simulink model "synchronized"  (R2018b)
settings: Solver=FixedStepAuto  StartTime=0.0  StopTime=0.1  FixedStep=0.0001  RelTol=1e-3
settings Model: Creator=User  LastModifiedBy=User

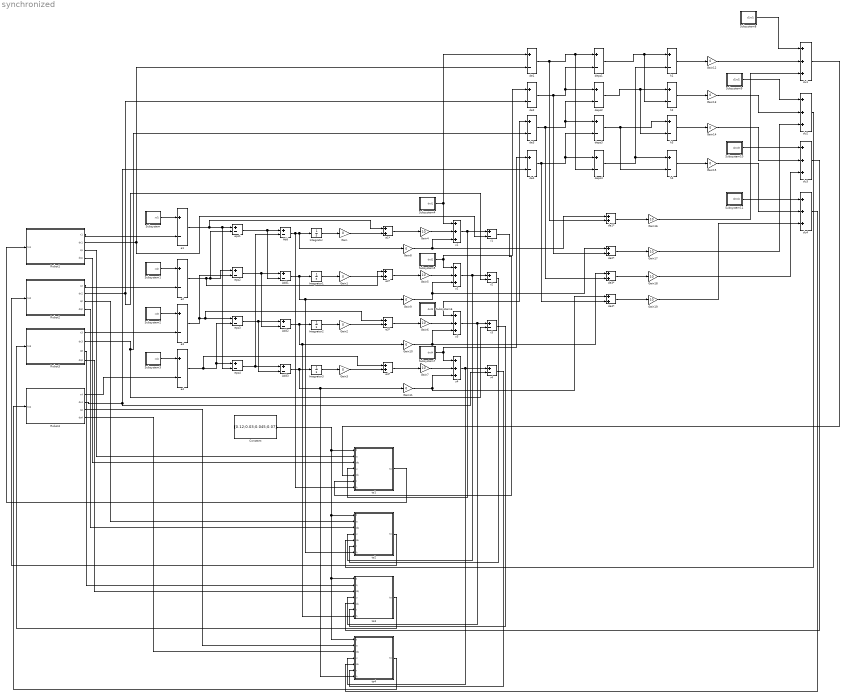
== system synchronized ==
  Add{,1..3} (4 alike) : Sum  Inputs=+-
  Constant : Constant  Value=[0.12;0.03;0.045;0.07]
  Gain{,1..3,8..15} (12 alike) : Gain  Gain=0
  Gain{4..7,16..19} (8 alike) : Gain  Gain=10
  Integrator{,1..3} (4 alike) : Integrator  InitialCondition=[0;0]
  Robot1 : Subsystem
  Robot2 : Subsystem
  Robot3 : Subsystem
  Robot4 : Subsystem
  Subsystem : Subsystem
  Subsystem1 : Subsystem
  Subsystem10 : Subsystem
  Subsystem11 : Subsystem
  Subsystem2 : Subsystem
  Subsystem3 : Subsystem
  Subsystem4 : Subsystem
  Subsystem5 : Subsystem
  Subsystem6 : Subsystem
  Subsystem7 : Subsystem
  Subsystem8 : Subsystem
  Subsystem9 : Subsystem
  de{1..4} (4 alike) : Sum  Inputs=+-
  de1* : Sum
  de2* : Sum
  de3* : Sum
  de4* : Sum
  deps{1..4} (4 alike) : Sum  Inputs=+-
  du{1..4} (4 alike) : Sum  Inputs=3
  e{1..4} (4 alike) : Sum  Inputs=+-
  e1* : Sum
  e2* : Sum
  e3* : Sum
  e4* : Sum
  eps{1..4} (4 alike) : Sum  Inputs=+-
  h{1..4} (4 alike) : Sum  Inputs=+-
  r{1..4} (4 alike) : Sum  Inputs=+-
  to1 : MATLAB Function  TreatAsAtomicUnit=on
  to2 : MATLAB Function  TreatAsAtomicUnit=on
  to3 : MATLAB Function  TreatAsAtomicUnit=on
  to4 : MATLAB Function  TreatAsAtomicUnit=on
  u{1..4} (4 alike) : Sum  Inputs=+++
  wires:
  Subsystem/1(xd1) -> e1/1
  Robot1/1(x1) -> e1/2
  Subsystem1/1(xd2) -> e2/1
  Robot2/1(x2) -> e2/2
  Robot3/1(x3) -> e3/2
  Subsystem2/1(xd3) -> e3/1
  Subsystem3/1(xd4) -> e4/1
  Robot4/1(x4) -> e4/2
  e1/1 -> e1*/1, eps4/2, eps1/1
  e2/1 -> e2*/1, eps1/2, eps2/1
  e3/1 -> e3*/1, eps3/1, eps2/2
  e4/1 -> e4*/1, eps4/1, eps3/2
  eps1/1 -> Add1/2, Add/1
  eps2/1 -> Add2/2, Add1/1
  eps3/1 -> Add2/1, Add3/2
  eps4/1 -> Add3/1, Add/2
  Add3/1 -> to4/7(h), Gain11/1, Integrator3/1
  Add2/1 -> to3/7(h), Gain10/1, Integrator2/1
  Add1/1 -> to2/7(h), Gain9/1, Integrator1/1
  Integrator/1 -> Gain/1
  Integrator1/1 -> Gain1/1
  Integrator2/1 -> Gain2/1
  Integrator3/1 -> Gain3/1
  Gain/1 -> e1*/2
  Gain1/1 -> e2*/2
  Gain2/1 -> e3*/2
  Gain3/1 -> e4*/2
  e1*/1 -> Gain4/1
  e4*/1 -> Gain7/1
  e3*/1 -> Gain6/1
  e2*/1 -> Gain5/1
  Subsystem4/1(dxd1) -> de1/1, u1/1
  Gain4/1 -> u1/2
  Gain8/1 -> de1*/1, u1/3
  Gain9/1 -> de2*/1, u2/3
  Gain5/1 -> u2/2
  Gain6/1 -> u3/2
  Gain10/1 -> de3*/1, u3/3
  Gain11/1 -> de4*/1, u4/3
  Gain7/1 -> u4/2
  Subsystem5/1(dxd2) -> de2/1, u2/1
  Subsystem6/1(dxd3) -> de3/1, u3/1
  Subsystem7/1(dxd4) -> de4/1, u4/1
  u4/1 -> to4/4(u), r4/1
  u3/1 -> to3/4(u), r3/1
  u2/1 -> to2/4(u), r2/1
  u1/1 -> to1/4(u), r1/1
  Robot1/2(dx1) -> r1/2, de1/2
  Robot2/2(dx2) -> r2/2, de2/2
  Robot3/2(dx3) -> de3/2, r3/2
  Robot4/2(dx4) -> de4/2, r4/2
  de1/1 -> de1*/2, deps4/2, deps1/1
  de2/1 -> de2*/2, deps2/1, deps1/2
  de3/1 -> de3*/2, deps3/1, deps2/2
  de4/1 -> de4*/2, deps4/1, deps3/2
  deps1/1 -> h2/2, h1/1
  deps4/1 -> h4/1, h1/2
  deps2/1 -> h3/2, h2/1
  deps3/1 -> h4/2, h3/1
  h1/1 -> Gain12/1
  h2/1 -> Gain13/1
  h3/1 -> Gain14/1
  h4/1 -> Gain15/1
  Gain12/1 -> du1/2
  Gain13/1 -> du2/2
  Gain14/1 -> du3/2
  Gain15/1 -> du4/2
  Subsystem8/1(d2xd1) -> du1/1
  Subsystem9/1(d2xd2) -> du2/1
  Subsystem10/1(d2xd3) -> du3/1
  Subsystem11/1(d2xd4) -> du4/1
  de4*/1 -> Gain19/1
  de3*/1 -> Gain18/1
  de2*/1 -> Gain17/1
  de1*/1 -> Gain16/1
  Gain16/1 -> du1/3
  Gain17/1 -> du2/3
  Gain18/1 -> du3/3
  Gain19/1 -> du4/3
  Robot1/3(q1) -> to1/2(q)
  Robot1/4(dq1) -> to1/3(dq)
  du1/1 -> to1/5(du)
  r1/1 -> to1/6(r)
  Add/1 -> to1/7(h), Gain8/1, Integrator/1
  Robot2/3(q2) -> to2/2(q)
  Robot2/4(dq2) -> to2/3(dq)
  Robot3/3(q3) -> to3/2(q)
  Robot3/4(dq3) -> to3/3(dq)
  Robot4/3(q4) -> to4/2(q)
  Robot4/4(dq4) -> to4/3(dq)
  r2/1 -> to2/6(r)
  r3/1 -> to3/6(r)
  r4/1 -> to4/6(r)
  du2/1 -> to2/5(du)
  du3/1 -> to3/5(du)
  du4/1 -> to4/5(du)
  to1/1(to) -> Robot1/1(to1)
  to2/1(to) -> Robot2/1(to2)
  to3/1(to) -> Robot3/1(to3)
  to4/1(to) -> Robot4/1(to4)
  Constant/1 -> to4/1(t), to3/1(t), to2/1(t), to1/1(t)

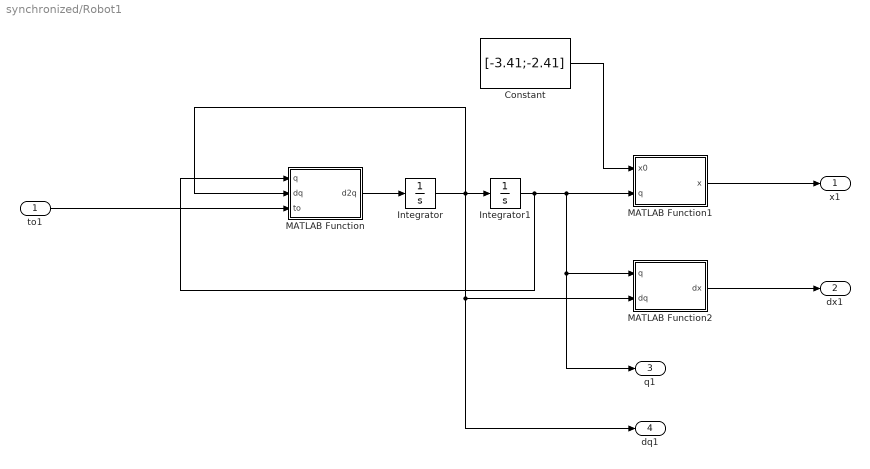
== system synchronized/Robot1 ==
  to1 : Inport
  Constant : Constant  Value=[-3.41;-2.41]
  Integrator : Integrator  InitialCondition=[0;0]
  Integrator1 : Integrator  InitialCondition=[pi/6;pi/6]
  MATLAB Function : MATLAB Function  TreatAsAtomicUnit=on
  MATLAB Function1 : MATLAB Function  TreatAsAtomicUnit=on
  MATLAB Function2 : MATLAB Function  TreatAsAtomicUnit=on
  x1 : Outport
  dx1 : Outport  Port=2
  q1 : Outport  Port=3
  dq1 : Outport  Port=4
  wires:
  to1/1 -> MATLAB Function/3(to)
  MATLAB Function/1(d2q) -> Integrator/1
  Integrator/1 -> dq1/1, MATLAB Function2/2(dq), MATLAB Function/2(dq), Integrator1/1
  Integrator1/1 -> q1/1, MATLAB Function2/1(q), MATLAB Function1/2(q), MATLAB Function/1(q)
  MATLAB Function1/1(x) -> x1/1
  Constant/1 -> MATLAB Function1/1(x0)
  MATLAB Function2/1(dx) -> dx1/1

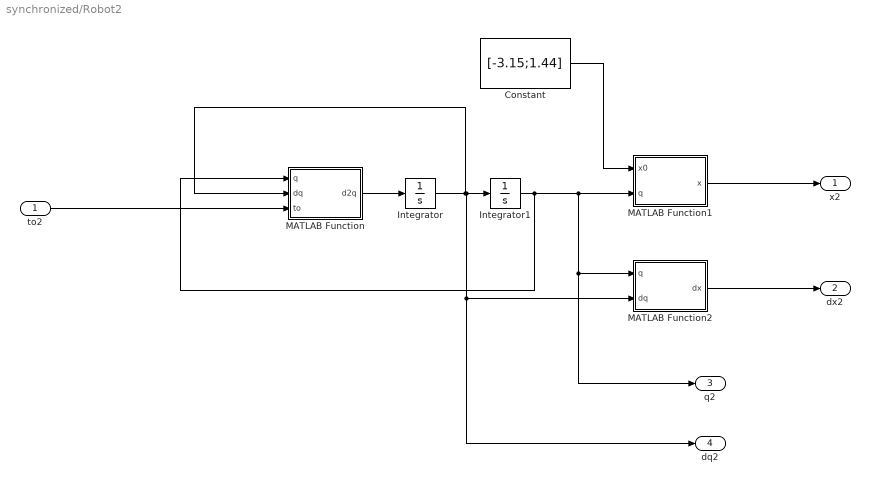
== system synchronized/Robot2 ==
  to2 : Inport
  Constant : Constant  Value=[-3.15;1.44]
  Integrator : Integrator  InitialCondition=[0;0]
  Integrator1 : Integrator  InitialCondition=[-0.37895;2.3932]
  MATLAB Function : MATLAB Function  TreatAsAtomicUnit=on
  MATLAB Function1 : MATLAB Function  TreatAsAtomicUnit=on
  MATLAB Function2 : MATLAB Function  TreatAsAtomicUnit=on
  x2 : Outport
  dx2 : Outport  Port=2
  q2 : Outport  Port=3
  dq2 : Outport  Port=4
  wires:
  Constant/1 -> MATLAB Function1/1(x0)
  MATLAB Function1/1(x) -> x2/1
  Integrator1/1 -> MATLAB Function/1(q), q2/1, MATLAB Function2/1(q), MATLAB Function1/2(q)
  Integrator/1 -> dq2/1, MATLAB Function2/2(dq), Integrator1/1, MATLAB Function/2(dq)
  MATLAB Function/1(d2q) -> Integrator/1
  to2/1 -> MATLAB Function/3(to)
  MATLAB Function2/1(dx) -> dx2/1

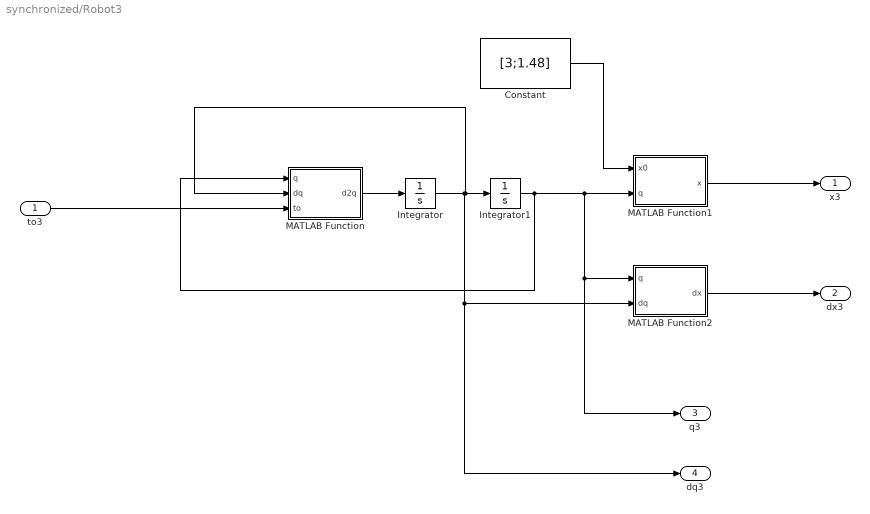
== system synchronized/Robot3 ==
  to3 : Inport
  Constant : Constant  Value=[3;1.48]
  Integrator : Integrator  InitialCondition=[0;0]
  Integrator1 : Integrator  InitialCondition=[-pi/6;pi/3]
  MATLAB Function : MATLAB Function  TreatAsAtomicUnit=on
  MATLAB Function1 : MATLAB Function  TreatAsAtomicUnit=on
  MATLAB Function2 : MATLAB Function  TreatAsAtomicUnit=on
  x3 : Outport
  dx3 : Outport  Port=2
  q3 : Outport  Port=3
  dq3 : Outport  Port=4
  wires:
  to3/1 -> MATLAB Function/3(to)
  MATLAB Function/1(d2q) -> Integrator/1
  Integrator/1 -> dq3/1, MATLAB Function2/2(dq), MATLAB Function/2(dq), Integrator1/1
  Integrator1/1 -> q3/1, MATLAB Function2/1(q), MATLAB Function1/2(q), MATLAB Function/1(q)
  MATLAB Function1/1(x) -> x3/1
  Constant/1 -> MATLAB Function1/1(x0)
  MATLAB Function2/1(dx) -> dx3/1

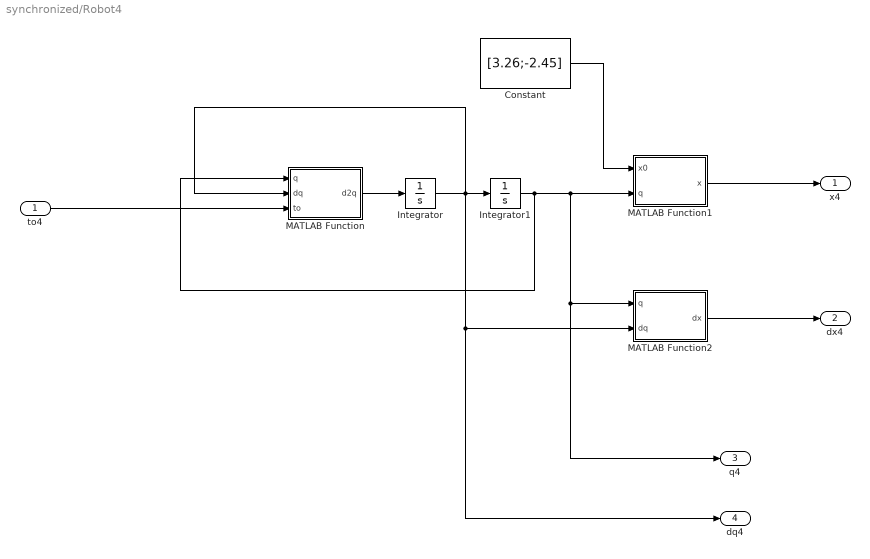
== system synchronized/Robot4 ==
  to4 : Inport
  Constant : Constant  Value=[3.26;-2.45]
  Integrator : Integrator  InitialCondition=[0;0]
  Integrator1 : Integrator  InitialCondition=[5*pi/6;-pi/3]
  MATLAB Function : MATLAB Function  TreatAsAtomicUnit=on
  MATLAB Function1 : MATLAB Function  TreatAsAtomicUnit=on
  MATLAB Function2 : MATLAB Function  TreatAsAtomicUnit=on
  x4 : Outport
  dx4 : Outport  Port=2
  q4 : Outport  Port=3
  dq4 : Outport  Port=4
  wires:
  Constant/1 -> MATLAB Function1/1(x0)
  MATLAB Function1/1(x) -> x4/1
  Integrator1/1 -> MATLAB Function/1(q), q4/1, MATLAB Function2/1(q), MATLAB Function1/2(q)
  Integrator/1 -> dq4/1, MATLAB Function2/2(dq), MATLAB Function/2(dq), Integrator1/1
  MATLAB Function/1(d2q) -> Integrator/1
  to4/1 -> MATLAB Function/3(to)
  MATLAB Function2/1(dx) -> dx4/1

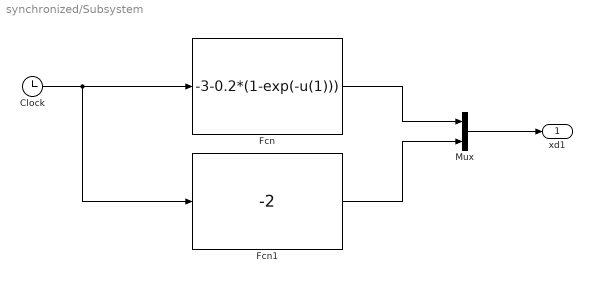
== system synchronized/Subsystem ==
  Clock : Clock
  Fcn : Fcn  Expr=-3-0.2*(1-exp(-u(1)))
  Fcn1 : Fcn  Expr=-2
  Mux : Mux  Inputs=2
  xd1 : Outport
  wires:
  Clock/1 -> Fcn1/1, Fcn/1
  Fcn/1 -> Mux/1
  Fcn1/1 -> Mux/2
  Mux/1 -> xd1/1

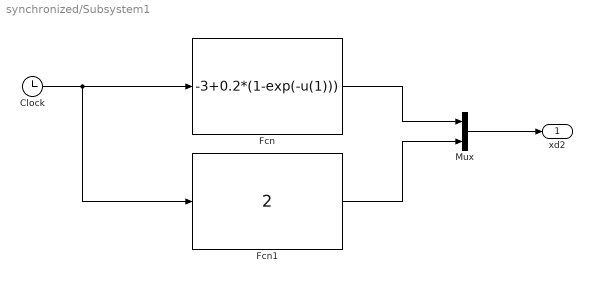
== system synchronized/Subsystem1 ==
  Clock : Clock
  Fcn : Fcn  Expr=-3+0.2*(1-exp(-u(1)))
  Fcn1 : Fcn  Expr=2
  Mux : Mux  Inputs=2
  xd2 : Outport
  wires:
  Mux/1 -> xd2/1
  Fcn1/1 -> Mux/2
  Fcn/1 -> Mux/1
  Clock/1 -> Fcn/1, Fcn1/1

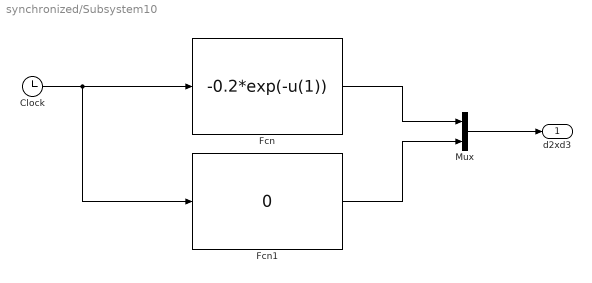
== system synchronized/Subsystem10 ==
  Clock : Clock
  Fcn : Fcn  Expr=-0.2*exp(-u(1))
  Fcn1 : Fcn  Expr=0
  Mux : Mux  Inputs=2
  d2xd3 : Outport
  wires:
  Clock/1 -> Fcn1/1, Fcn/1
  Fcn/1 -> Mux/1
  Fcn1/1 -> Mux/2
  Mux/1 -> d2xd3/1

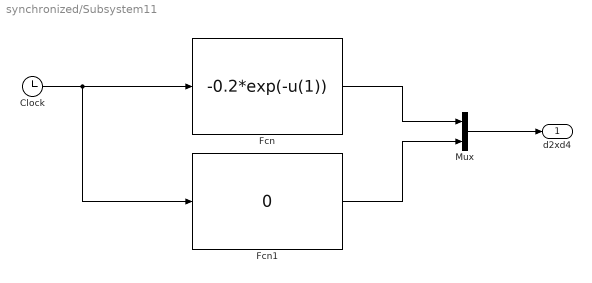
== system synchronized/Subsystem11 ==
  Clock : Clock
  Fcn : Fcn  Expr=-0.2*exp(-u(1))
  Fcn1 : Fcn  Expr=0
  Mux : Mux  Inputs=2
  d2xd4 : Outport
  wires:
  Mux/1 -> d2xd4/1
  Fcn1/1 -> Mux/2
  Fcn/1 -> Mux/1
  Clock/1 -> Fcn/1, Fcn1/1

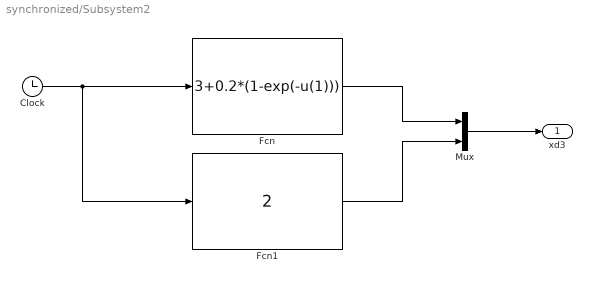
== system synchronized/Subsystem2 ==
  Clock : Clock
  Fcn : Fcn  Expr=3+0.2*(1-exp(-u(1)))
  Fcn1 : Fcn  Expr=2
  Mux : Mux  Inputs=2
  xd3 : Outport
  wires:
  Clock/1 -> Fcn1/1, Fcn/1
  Fcn/1 -> Mux/1
  Fcn1/1 -> Mux/2
  Mux/1 -> xd3/1

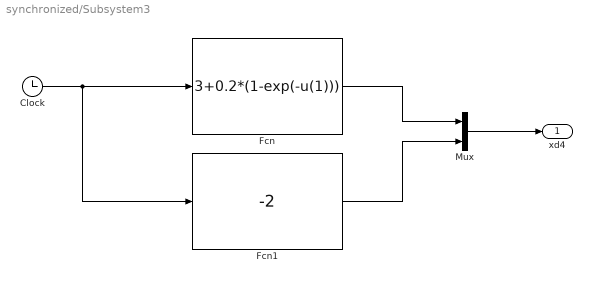
== system synchronized/Subsystem3 ==
  Clock : Clock
  Fcn : Fcn  Expr=3+0.2*(1-exp(-u(1)))
  Fcn1 : Fcn  Expr=-2
  Mux : Mux  Inputs=2
  xd4 : Outport
  wires:
  Mux/1 -> xd4/1
  Fcn1/1 -> Mux/2
  Fcn/1 -> Mux/1
  Clock/1 -> Fcn/1, Fcn1/1

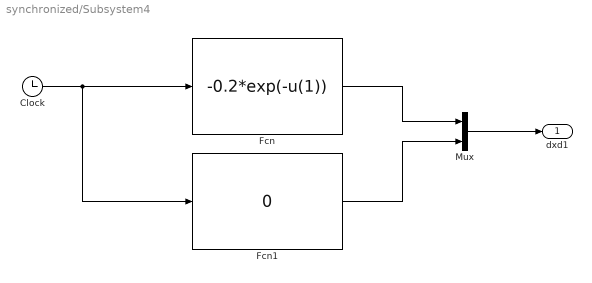
== system synchronized/Subsystem4 ==
  Clock : Clock
  Fcn : Fcn  Expr=-0.2*exp(-u(1))
  Fcn1 : Fcn  Expr=0
  Mux : Mux  Inputs=2
  dxd1 : Outport
  wires:
  Mux/1 -> dxd1/1
  Fcn1/1 -> Mux/2
  Fcn/1 -> Mux/1
  Clock/1 -> Fcn/1, Fcn1/1

== system synchronized/Subsystem5 ==
  Clock : Clock
  Fcn : Fcn  Expr=0.2*exp(-u(1))
  Fcn1 : Fcn  Expr=0
  Mux : Mux  Inputs=2
  dxd2 : Outport
  wires:
  Clock/1 -> Fcn1/1, Fcn/1
  Fcn/1 -> Mux/1
  Fcn1/1 -> Mux/2
  Mux/1 -> dxd2/1

== system synchronized/Subsystem6 ==
  Clock : Clock
  Fcn : Fcn  Expr=0.2*exp(-u(1))
  Fcn1 : Fcn  Expr=0
  Mux : Mux  Inputs=2
  dxd3 : Outport
  wires:
  Mux/1 -> dxd3/1
  Fcn1/1 -> Mux/2
  Fcn/1 -> Mux/1
  Clock/1 -> Fcn/1, Fcn1/1

== system synchronized/Subsystem7 ==
  Clock : Clock
  Fcn : Fcn  Expr=0.2*exp(-u(1))
  Fcn1 : Fcn  Expr=0
  Mux : Mux  Inputs=2
  dxd4 : Outport
  wires:
  Clock/1 -> Fcn1/1, Fcn/1
  Fcn/1 -> Mux/1
  Fcn1/1 -> Mux/2
  Mux/1 -> dxd4/1

== system synchronized/Subsystem8 ==
  Clock : Clock
  Fcn : Fcn  Expr=0.2*exp(-u(1))
  Fcn1 : Fcn  Expr=0
  Mux : Mux  Inputs=2
  d2xd1 : Outport
  wires:
  Clock/1 -> Fcn1/1, Fcn/1
  Fcn/1 -> Mux/1
  Fcn1/1 -> Mux/2
  Mux/1 -> d2xd1/1

== system synchronized/Subsystem9 ==
  Clock : Clock
  Fcn : Fcn  Expr=-0.2*exp(-u(1))
  Fcn1 : Fcn  Expr=0
  Mux : Mux  Inputs=2
  d2xd2 : Outport
  wires:
  Mux/1 -> d2xd2/1
  Fcn1/1 -> Mux/2
  Fcn/1 -> Mux/1
  Clock/1 -> Fcn/1, Fcn1/1

== matlab function synchronized/Robot1/MATLAB Function1 ==
  data: x0 input; x output; q input
function x = fcn(x0,q)
q1=q(1);
q2=q(2);
x=x0+[0.3*cos(q1)+0.3*cos(q1+q2);0.3*sin(q1)+0.3*sin(q1+q2)];
end

== matlab function synchronized/Robot1/MATLAB Function ==
  data: q input; d2q output; dq input; to input
function d2q = fcn(q,dq,to)
m1=1;
m2=1;
l1=0.3;
l2=0.3;
t1=1/3*m1*l1^2+m2*l1^2;
t2=1/3*m2*l2^2;
t3=1/2*m2*l1*l2;
t4=0.07;
q2=q(2);
M=[t1+t2+2*t3*cos(q2) t2+t3*cos(q2);
    t2+t3*cos(q2) t2];
dq1=dq(1);
dq2=dq(2);
V=[-dq2*dq1*t3*sin(q2)-(dq1+dq2)*dq2*t3*sin(q2)+t4*dq1;
    dq1^2*t3*sin(q2)+t4*dq2];
d2q=M\(to-V);
end

== matlab function synchronized/Robot2/MATLAB Function ==
  data: q input; d2q output; dq input; to input
function d2q = fcn(q,dq,to)
m1=1;
m2=1;
l1=0.3;
l2=0.3;
t1=1/3*m1*l1^2+m2*l1^2;
t2=1/3*m2*l2^2;
t3=1/2*m2*l1*l2;
t4=0.07;
q2=q(2);
M=[t1+t2+2*t3*cos(q2) t2+t3*cos(q2);
    t2+t3*cos(q2) t2];
dq1=dq(1);
dq2=dq(2);
V=[-dq2*dq1*t3*sin(q2)-(dq1+dq2)*dq2*t3*sin(q2)+t4*dq1;
    dq1^2*t3*sin(q2)+t4*dq2];
d2q=M\(to-V);
end

== matlab function synchronized/Robot2/MATLAB Function1 ==
  data: x0 input; x output; q input
function x = fcn(x0,q)
q1=q(1);
q2=q(2);
x=x0+[0.3*cos(q1)+0.3*cos(q1+q2);0.3*sin(q1)+0.3*sin(q1+q2)];
end

== matlab function synchronized/Robot3/MATLAB Function ==
  data: q input; d2q output; dq input; to input
function d2q = fcn(q,dq,to)
m1=1;
m2=1;
l1=0.3;
l2=0.3;
t1=1/3*m1*l1^2+m2*l1^2;
t2=1/3*m2*l2^2;
t3=1/2*m2*l1*l2;
t4=0.07;
q2=q(2);
M=[t1+t2+2*t3*cos(q2) t2+t3*cos(q2);
    t2+t3*cos(q2) t2];
dq1=dq(1);
dq2=dq(2);
V=[-dq2*dq1*t3*sin(q2)-(dq1+dq2)*dq2*t3*sin(q2)+t4*dq1;
    dq1^2*t3*sin(q2)+t4*dq2];
d2q=M\(to-V);
end

== matlab function synchronized/Robot3/MATLAB Function1 ==
  data: x0 input; x output; q input
function x = fcn(x0,q)
q1=q(1);
q2=q(2);
x=x0+[0.3*cos(q1)+0.3*cos(q1+q2);0.3*sin(q1)+0.3*sin(q1+q2)];
end

== matlab function synchronized/Robot4/MATLAB Function ==
  data: q input; d2q output; dq input; to input
function d2q = fcn(q,dq,to)
m1=1;
m2=1;
l1=0.3;
l2=0.3;
t1=1/3*m1*l1^2+m2*l1^2;
t2=1/3*m2*l2^2;
t3=1/2*m2*l1*l2;
t4=0.07;
q2=q(2);
M=[t1+t2+2*t3*cos(q2) t2+t3*cos(q2);
    t2+t3*cos(q2) t2];
dq1=dq(1);
dq2=dq(2);
V=[-dq2*dq1*t3*sin(q2)-(dq1+dq2)*dq2*t3*sin(q2)+t4*dq1;
    dq1^2*t3*sin(q2)+t4*dq2];
d2q=M\(to-V);
end

== matlab function synchronized/Robot4/MATLAB Function1 ==
  data: x0 input; x output; q input
function x = fcn(x0,q)
q1=q(1);
q2=q(2);
x=x0+[0.3*cos(q1)+0.3*cos(q1+q2);0.3*sin(q1)+0.3*sin(q1+q2)];
end

== matlab function synchronized/Robot1/MATLAB Function2 ==
  data: q input; dq input; dx output
function dx = fcn(q,dq)
q1=q(1);
q2=q(2);
J=[-0.3*sin(q1)-0.3*sin(q1+q2) -0.3*sin(q1+q2);
    0.3*cos(q1)+0.3*cos(q1+q2) 0.3*cos(q1+q2)];
dx=J*dq;
end

== matlab function synchronized/Robot2/MATLAB Function2 ==
  data: q input; dq input; dx output
function dx = fcn(q,dq)
q1=q(1);
q2=q(2);
J=[-0.3*sin(q1)-0.3*sin(q1+q2) -0.3*sin(q1+q2);
    0.3*cos(q1)+0.3*cos(q1+q2) 0.3*cos(q1+q2)];
dx=J*dq;
end

== matlab function synchronized/Robot3/MATLAB Function2 ==
  data: q input; dq input; dx output
function dx = fcn(q,dq)
q1=q(1);
q2=q(2);
J=[-0.3*sin(q1)-0.3*sin(q1+q2) -0.3*sin(q1+q2);
    0.3*cos(q1)+0.3*cos(q1+q2) 0.3*cos(q1+q2)];
dx=J*dq;
end

== matlab function synchronized/Robot4/MATLAB Function2 ==
  data: q input; dq input; dx output
function dx = fcn(q,dq)
q1=q(1);
q2=q(2);
J=[-0.3*sin(q1)-0.3*sin(q1+q2) -0.3*sin(q1+q2);
    0.3*cos(q1)+0.3*cos(q1+q2) 0.3*cos(q1+q2)];
dx=J*dq;
end

== matlab function synchronized/to1 ==
  data: t input; q input; dq input; u input; to output; du input; r input; h input
function to = fcn(t,q,dq,u,du,r,h)
t1=t(1);
t2=t(2);
t3=t(3);
t4=t(4);
q1=q(1);
q2=q(2);
Hq=[t1+t2+2*t3*cos(q2) t2+t3*cos(q2);
    t2+t3*cos(q2) t2];
dq1=dq(1);
dq2=dq(2);
Cq=[-dq2*t3*sin(q2) -(dq1+dq2)*t3*sin(q2);
    dq1*t3*sin(q2) 0];
Fq=[t4*dq1;t4*dq2];
J=[-0.3*sin(q1)-0.3*sin(q1+q2) -0.3*sin(q1+q2);
    0.3*cos(q1)+0.3*cos(q1+q2) 0.3*cos(q1+q2)];
dJ=[-0.3*dq1*cos(q1)-0.3*(dq1+dq2)*cos(q1+q2) -0.3*(dq1+dq2)*cos(q1+q2);
    -0.3*dq1*sin(q1)-0.3*(dq1+dq2)*sin(q1+q2) -0.3*(dq1+dq2)*sin(q1+q2)];
Hx=Hq/J;
Cx=Cq/J-(Hq/J)*(dJ/J);
to=Hx*du+Cx*u+Fq+1*r+0*h;
end

== matlab function synchronized/to2 ==
  data: t input; q input; dq input; u input; to output; du input; r input; h input
function to = fcn(t,q,dq,u,du,r,h)
t1=t(1);
t2=t(2);
t3=t(3);
t4=t(4);
q1=q(1);
q2=q(2);
Hq=[t1+t2+2*t3*cos(q2) t2+t3*cos(q2);
    t2+t3*cos(q2) t2];
dq1=dq(1);
dq2=dq(2);
Cq=[-dq2*t3*sin(q2) -(dq1+dq2)*t3*sin(q2);
    dq1*t3*sin(q2) 0];
Fq=[t4*dq1;t4*dq2];
J=[-0.3*sin(q1)-0.3*sin(q1+q2) -0.3*sin(q1+q2);
    0.3*cos(q1)+0.3*cos(q1+q2) 0.3*cos(q1+q2)];
dJ=[-0.3*dq1*cos(q1)-0.3*(dq1+dq2)*cos(q1+q2) -0.3*(dq1+dq2)*cos(q1+q2);
    -0.3*dq1*sin(q1)-0.3*(dq1+dq2)*sin(q1+q2) -0.3*(dq1+dq2)*sin(q1+q2)];
Hx=Hq/J;
Cx=Cq/J-(Hq/J)*(dJ/J);
to=Hx*du+Cx*u+Fq+1*r+0*h;
end

== matlab function synchronized/to3 ==
  data: t input; q input; dq input; u input; to output; du input; r input; h input
function to = fcn(t,q,dq,u,du,r,h)
t1=t(1);
t2=t(2);
t3=t(3);
t4=t(4);
q1=q(1);
q2=q(2);
Hq=[t1+t2+2*t3*cos(q2) t2+t3*cos(q2);
    t2+t3*cos(q2) t2];
dq1=dq(1);
dq2=dq(2);
Cq=[-dq2*t3*sin(q2) -(dq1+dq2)*t3*sin(q2);
    dq1*t3*sin(q2) 0];
Fq=[t4*dq1;t4*dq2];
J=[-0.3*sin(q1)-0.3*sin(q1+q2) -0.3*sin(q1+q2);
    0.3*cos(q1)+0.3*cos(q1+q2) 0.3*cos(q1+q2)];
dJ=[-0.3*dq1*cos(q1)-0.3*(dq1+dq2)*cos(q1+q2) -0.3*(dq1+dq2)*cos(q1+q2);
    -0.3*dq1*sin(q1)-0.3*(dq1+dq2)*sin(q1+q2) -0.3*(dq1+dq2)*sin(q1+q2)];
Hx=Hq/J;
Cx=Cq/J-(Hq/J)*(dJ/J);
to=Hx*du+Cx*u+Fq+1*r+0*h;
end

== matlab function synchronized/to4 ==
  data: t input; q input; dq input; u input; to output; du input; r input; h input
function to = fcn(t,q,dq,u,du,r,h)
t1=t(1);
t2=t(2);
t3=t(3);
t4=t(4);
q1=q(1);
q2=q(2);
Hq=[t1+t2+2*t3*cos(q2) t2+t3*cos(q2);
    t2+t3*cos(q2) t2];
dq1=dq(1);
dq2=dq(2);
Cq=[-dq2*t3*sin(q2) -(dq1+dq2)*t3*sin(q2);
    dq1*t3*sin(q2) 0];
Fq=[t4*dq1;t4*dq2];
J=[-0.3*sin(q1)-0.3*sin(q1+q2) -0.3*sin(q1+q2);
    0.3*cos(q1)+0.3*cos(q1+q2) 0.3*cos(q1+q2)];
dJ=[-0.3*dq1*cos(q1)-0.3*(dq1+dq2)*cos(q1+q2) -0.3*(dq1+dq2)*cos(q1+q2);
    -0.3*dq1*sin(q1)-0.3*(dq1+dq2)*sin(q1+q2) -0.3*(dq1+dq2)*sin(q1+q2)];
Hx=Hq/J;
Cx=Cq/J-(Hq/J)*(dJ/J);
to=Hx*du+Cx*u+Fq+1*r+0*h;
end
